simulink model "stateflowPractice"  (R2023b)
settings: Solver=FixedStepAuto  StartTime=0.0  StopTime=inf  RelTol=1e-3  EnableMultiTasking=on
libraries: vexarmcortexlib x3
settings Model: Creator=behja  LastModifiedBy=behja
settings DataIOCC: LimitDataPoints=on  SignalLoggingSaveFormat=ModelDataLogs  ReturnWorkspaceOutputs=off
settings OptimizationCC: ExpressionDepthLimit=2147483647  LifeSpan=Inf  MaxStackSize=64  EfficientTunableParamExpr=on
settings DebuggingCC: UnderspecifiedInitializationDetection=Classic  MergeDetectMultiDrivingBlocksExec=none  InheritedTsInSrcMsg=none  FcnCallInpInsideContextMsg=warning  StateNameClashWarn=warning  SFUnexpectedBacktrackingDiag=warning  SFNoUnconditionalDefaultTransitionDiag=warning  SFExecutionAtInitializationDiag=none  ArithmeticOperatorsInVariantConditions=warning
settings HardwareCC: ProdBitPerPointer=32  ProdBitPerSizeT=32  ProdBitPerPtrDiffT=32  ProdLargestAtomicInteger=Long  ProdLargestAtomicFloat=Double  ProdIntDivRoundTo=Undefined  ProdWordSize=32  ProdHWDeviceType=ARM Compatible->ARM Cortex
settings ModelReferenceCC: EnableRefExpFcnMdlSchedulingChecks=on  PropagateSignalLabelsOutOfModel=off
settings SFSimCC: MATLABDynamicMemAlloc=off  CustomCodeUndefinedFunction=UseInterfaceOnly
settings RTWCC: Description=Embedded Coder  SystemTargetFile=ert.tlc  HardwareBoard=ARM Cortex-based VEX Microcontroller  TemplateMakefile=ert_default_tmf  Toolchain=GNU Tools for VEX ARM Cortex
settings CodeAppCC: IgnoreCustomStorageClasses=off  CustomSymbolStrType=$N$R$M  StateflowObjectComments=on  InternalIdentifier=Classic
settings ERTTargetCC: CodeReplacementLibrary=GCC ARM Cortex-M3  MultiwordLength=2048  ConvertIfToSwitch=off  SuppressUnreachableDefaultCases=off

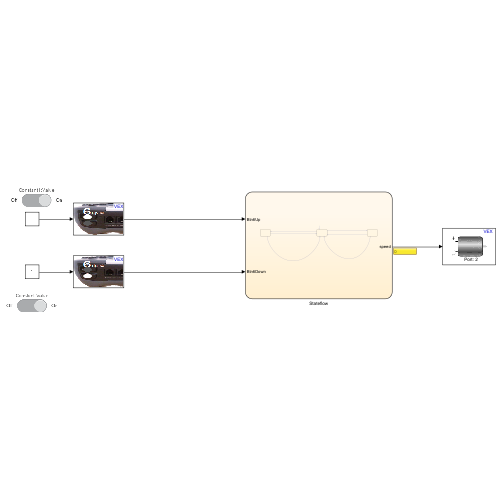
[thumbnail: Simulink's stored preview of the top-level diagram]
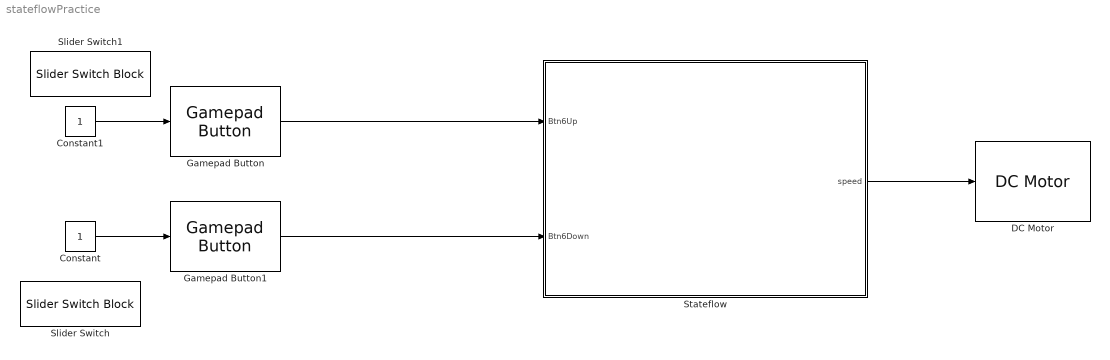
== system stateflowPractice ==
  Constant : Constant
  Constant1 : Constant
  DC Motor : vexarmcortexlib/Actuators/DC Motor  motor=2  scaleFactor=1/13.5  SimulationOut=off
  Gamepad Button : vexarmcortexlib/Gamepad/Gamepad Button  joystick=1  chan=6  button56=Up  button78=Down  SimulationIn=on  SampleTime=0.02
  Gamepad Button1 : vexarmcortexlib/Gamepad/Gamepad Button  joystick=1  chan=6  button56=Down  button78=Down  SimulationIn=on  SampleTime=0.02
  Slider Switch : SliderSwitchBlock
      settings: Values={{'Off', 'On'}, [0 1]}
  Slider Switch1 : SliderSwitchBlock
      settings: Values={{'Off', 'On'}, [0 1]}
  Stateflow : Stateflow chart  TreatAsAtomicUnit=on
  wires:
  Constant/1 -> Gamepad Button1/1
  Constant1/1 -> Gamepad Button/1
  Gamepad Button/1 -> Stateflow/1(Btn6Up)
  Gamepad Button1/1 -> Stateflow/2(Btn6Down)
  Stateflow/1(speed) -> DC Motor/1

== stateflow chart stateflowPractice/Stateflow ==
  state ArmDOWN
    entry:
    speed=-127;
  state STOPPED
    entry:
    speed=0;
  state ArmUP
    entry:
    speed=127;
  (default) -> STOPPED
  STOPPED -> ArmUP [order 2] : [Btn6Down==0 && Btn6Up==1]
  STOPPED -> ArmDOWN [order 1] : [Btn6Down==1 && Btn6Up==0]
  ArmDOWN -> STOPPED [order 1] : [Btn6Down==0]
  ArmUP -> STOPPED [order 1] : [Btn6Up==0]
  ArmDOWN -> STOPPED [order 2] : [Btn6Down==1 && Btn6Up==1]
  ArmUP -> STOPPED [order 2] : [Btn6Down==1 && Btn6Up==1]
  data: speed output; Btn6Up input; Btn6Down input
